simulink model "Lab45"  (R2020b)
settings: Solver=VariableStepAuto  StartTime=0.0  StopTime=10.0  RelTol=1e-3
model workspace (MAT data in the model file):
  u = Simulink.Parameter
  u.DataType = 'auto'
  u.Dimensions = [0 0]
libraries: simulink x1
settings Model: Creator=evpet  LastModifiedBy=evpet

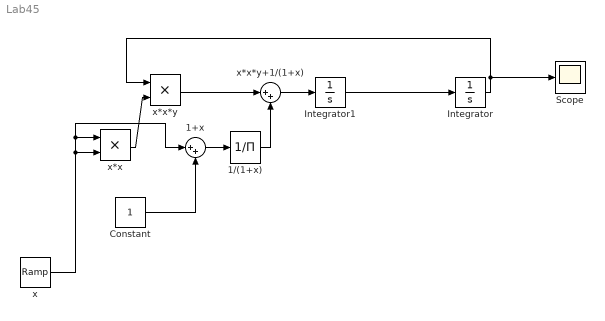
== system Lab45 ==
  1+x : Sum  Inputs=|++
  1/(1+x) : Product  Inputs=/
  Constant : Constant
  Integrator : Integrator
  Integrator1 : Integrator
  Scope : Scope
  x : simulink/Sources/Ramp  slope=1  start=0  InitialOutput=0
  x*x : Product
  x*x*y : Product
  x*x*y+1/(1+x) : Sum  Inputs=|++
  wires:
  x/1 -> x*x/1, 1+x/1, x*x/2
  x*x/1 -> x*x*y/2
  Integrator1/1 -> Integrator/1
  Integrator/1 -> x*x*y/1, Scope/1
  Constant/1 -> 1+x/2
  1+x/1 -> 1/(1+x)/1
  x*x*y/1 -> x*x*y+1/(1+x)/1
  1/(1+x)/1 -> x*x*y+1/(1+x)/2
  x*x*y+1/(1+x)/1 -> Integrator1/1
